simulink model "sldemo_mdlref_counter_datamngt"  (Simulink 7.6)
settings: Solver=FixedStepDiscrete  StartTime=0.0  StopTime=10.0  FixedStep=Auto  RelTol=1e-3  SampleTimeConstraint=STIndependent
PreLoadFcn:
  | sldemo_mdlref_counter_datamngt_types
model workspace (MATLAB code in the model file):
  | sldemo_mdlref_counter_datamngt_wsdata
undefined symbols (not defined in the file or in its folder): CounterICs, CounterParams
settings Model: Creator=The MathWorks Inc.  ExtModeAutoUpdateStatusClock=off
settings DataIOCC: SaveFormat=StructureWithTime  SaveOutput=off  SignalLogging=off  DSMLogging=off  SaveTime=off  SignalLoggingName=logsOut
settings OptimizationCC: InlineParams=on  InlineInvariantSignals=on  EnhancedBackFolding=on  StrengthReduction=on  StateBitsets=on  DataBitsets=on  UseTempVars=on  EfficientFloat2IntCast=on
settings DebuggingCC: SaveWithParameterizedLinksMsg=none  UnderspecifiedInitializationDetection=Simplified  CheckExecutionContextPreStartOutputMsg=on  CheckExecutionContextRuntimeOutputMsg=on  SolverPrmCheckMsg=none  MultiTaskDSMMsg=warning  MultiTaskCondExecSysMsg=none  SigSpecEnsureSampleTimeMsg=none  StrictBusMsg=ErrorOnBusTreatedAsVector
settings HardwareCC: TargetHWDeviceType=32-bit Generic
settings ModelReferenceCC: UpdateModelReferenceTargets=IfOutOfDate  CheckModelReferenceTargetMessage=none
settings SFSimCC: SimParseCustomCode=off
settings RTWCC: GenerateReport=on  RTWVerbose=off  ProcessScript=grt_make_rtw_hook  LaunchReport=on  IncludeERTFirstTime=on
settings CodeAppCC: ForceParamTrailComments=on  MaxIdLength=100
settings GRTTargetCC: MatFileLogging=off

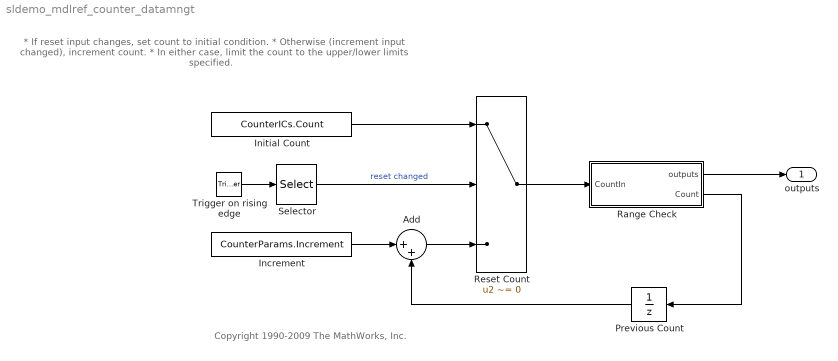
== system sldemo_mdlref_counter_datamngt ==
  note: Copyright 1990-2009 The MathWorks, Inc.
  note: * If reset input changes, set count to initial condition.
      | * Otherwise (increment input changed), increment count.
      | * In either case, limit the count to the upper/lower limits specified.
  Trigger on rising edge : TriggerPort  ShowOutputPort=on  OutputDataType=int8  PortDimensions=2  OutDataTypeStr=boolean  Interpolate=off
  Add : Sum  Inputs=|++  OutDataTypeStr=int8
  Increment : Constant  Value=CounterParams.Increment
  Initial Count : Constant  Value=CounterICs.Count
  Previous Count : UnitDelay  X0=CounterICs.Count  SampleTime=-1  StateIdentifier=PrevCount
  Range Check : Subsystem
  Reset Count : Switch  Criteria=u2 ~= 0
  Selector : Selector  InputPortWidth=2  IndexOptions=Index vector (dialog)  Indices=1  OutputSizes=1
  outputs : Outport  OutDataTypeStr=Bus: OutputType  InitialOutput=CounterICs  BusOutputAsStruct=on
  wires:
  Reset Count/1 -> Range Check/1(CountIn)
  Initial Count/1 -> Reset Count/1
  Previous Count/1 -> Add/2
  Range Check/1(outputs) -> outputs/1
  Range Check/2(Count) -> Previous Count/1
  Trigger on rising edge/1 -> Selector/1
  Selector/1 -> Reset Count/2  "reset changed"
  Add/1 -> Reset Count/3
  Increment/1 -> Add/1

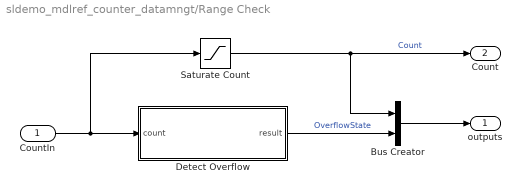
== system sldemo_mdlref_counter_datamngt/Range Check ==
  CountIn : Inport
  Bus Creator : BusCreator  Inputs=2  OutDataTypeStr=Bus: OutputType  NonVirtualBus=on
  Detect Overflow : Stateflow chart  TreatAsAtomicUnit=on
  Saturate Count : Saturate  UpperLimit=CounterParams.UpperLimit  LowerLimit=CounterParams.LowerLimit
  outputs : Outport
  Count : Outport  Port=2
  wires:
  CountIn/1 -> Saturate Count/1, Detect Overflow/1(count)
  Saturate Count/1 -> Count/1, Bus Creator/1  "Count"
  Detect Overflow/1(result) -> Bus Creator/2  "OverflowState"
  Bus Creator/1 -> outputs/1

== matlab function Range Check/Detect Overflow ==
  data: count input double; result output double; CounterParams parameter double
function result = DetectOverflow(count, CounterParams)
% DETECTOVERFLOW  Check count
%#eml

if (count >= CounterParams.UpperLimit)
  result = SlDemoRangeCheck.UpperLimit;
elseif (count > CounterParams.LowerLimit)
  result = SlDemoRangeCheck.InRange;
else
  result = SlDemoRangeCheck.LowerLimit;
end
